simulink model "observer_student"  (R2020b)
settings: Solver=FixedStepAuto  StartTime=0.0  StopTime=Inf  RelTol=1e-3
undefined symbols (not defined in the file): X, Y, Z
libraries: robotlib x12
settings Model: Creator=erlendbasso  LastModifiedBy=erlendbasso
settings OptimizationCC: EnhancedBackFolding=on  PassReuseOutputArgsAs=Individual arguments  ZeroExternalMemoryAtStartup=off  ZeroInternalMemoryAtStartup=off  MaxStackSize=64  OptimizeBlockOrder=speed  DifferentSizesBufferReuse=on  OptimizationCustomize=off  EfficientTunableParamExpr=on
settings DebuggingCC: ParameterTunabilityLossMsg=error
settings HardwareCC: ProdBitPerPointer=32  ProdBitPerSizeT=32  ProdBitPerPtrDiffT=32  ProdLargestAtomicInteger=Long  ProdLargestAtomicFloat=Double  ProdWordSize=32  ProdHWDeviceType=ARM Compatible->ARM Cortex
settings RTWCC: Description=Embedded Coder  SystemTargetFile=ert.tlc  HardwareBoard=Raspberry Pi - Robot Operating System (ROS)  TLCOptions="-aInlineSetEventsForThisBaseRateFcn=TLC_FALSE -aSuppressMultiTaskScheduler=TLC_FALSE  -aRateBasedStepFcn=0"  TemplateMakefile=ert_default_tmf  Toolchain=Catkin  TargetLang=C++
settings CodeAppCC: ForceParamTrailComments=on  IgnoreCustomStorageClasses=off  OperatorAnnotations=on  SimulinkDataObjDesc=on  SFDataObjDesc=on  InsertBlockDesc=on
settings ERTTargetCC: SupportContinuousTime=on  SupportVariableSizeSignals=on

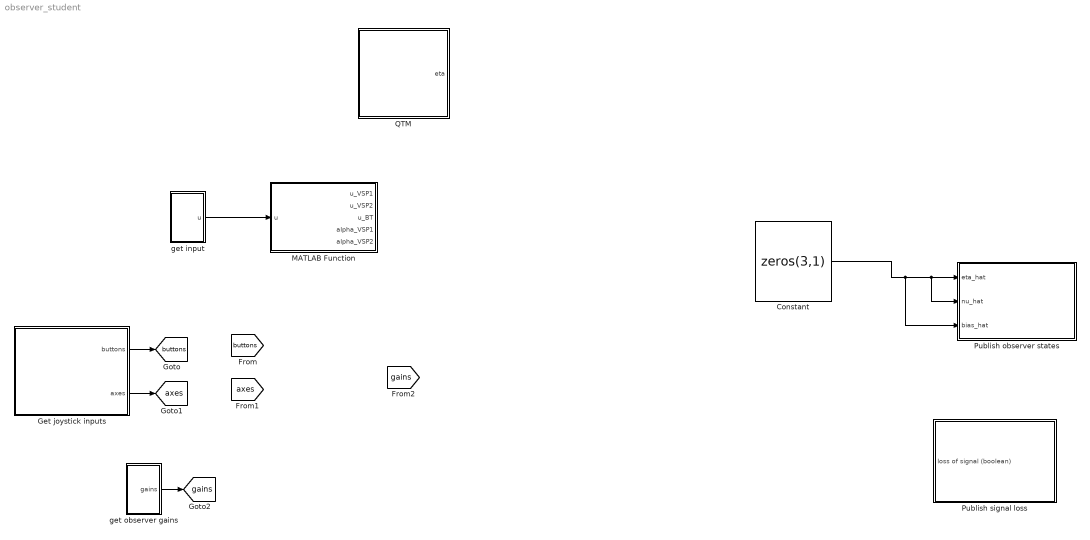
== system observer_student ==
  Constant : Constant  Value=zeros(3,1)
  Get joystick inputs : Subsystem
  MATLAB Function : MATLAB Function  TreatAsAtomicUnit=on
  Publish observer states : Subsystem
  Publish signal loss : Subsystem
  QTM : Subsystem
  get input : Subsystem
  get observer gains : Subsystem
  tag scope: axes=global, buttons=global, gains=global
  wires:
  get input/1(u) -> MATLAB Function/1(u)
  Constant/1 -> Publish observer states/3(bias_hat), Publish observer states/2(nu_hat), Publish observer states/1(eta_hat)
  Get joystick inputs/2(axes) -> [axes]
  Get joystick inputs/1(buttons) -> [buttons]
  get observer gains/1(gains) -> [gains]

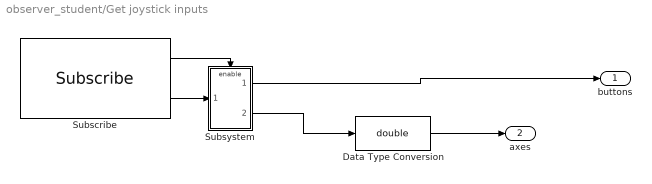
== system observer_student/Get joystick inputs ==
  Data Type Conversion : DataTypeConversion  OutDataTypeStr=double
  Subscribe : robotlib/Subscribe  topicSource=Select from ROS network  topic=/joy  messageType=sensor_msgs/Joy  SampleTime=0.01  legacyBusStruct=off  messageQueueLength=1
  Subsystem : Subsystem
  buttons : Outport
  axes : Outport  Port=2
  wires:
  Subscribe/1 -> Subsystem/Enable
  Subscribe/2 -> Subsystem/1(In1)
  Subsystem/2(<Axes>) -> Data Type Conversion/1
  Subsystem/1(<Buttons>) -> buttons/1
  Data Type Conversion/1 -> axes/1

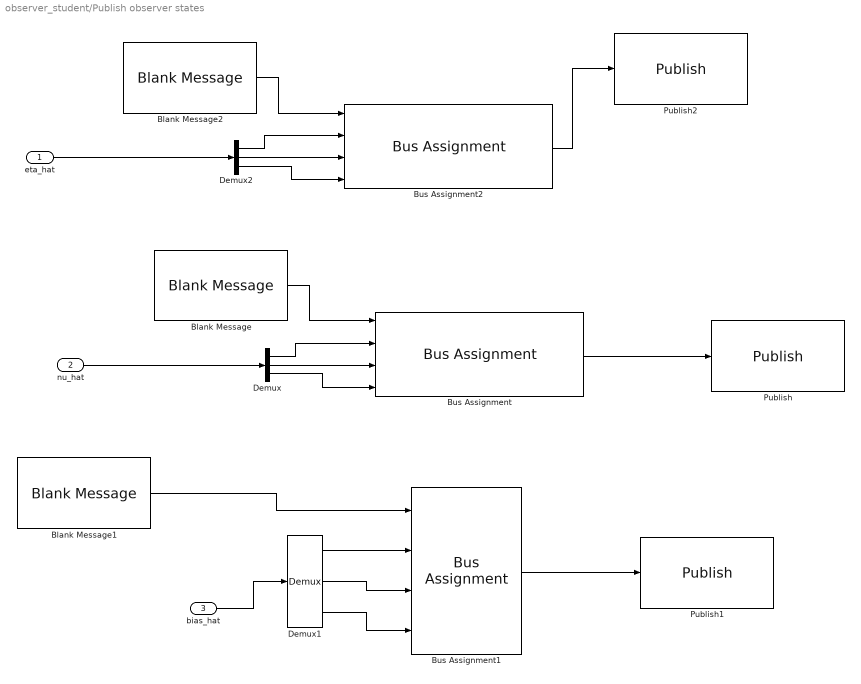
== system observer_student/Publish observer states ==
  eta_hat : Inport
  nu_hat : Inport  Port=2
  bias_hat : Inport  Port=3
  Blank Message : robotlib/Blank Message  messageClass=Message  entityType=geometry_msgs/Vector3  messageType=geometry_msgs/Vector3  SampleTime=0.01  legacyBusStruct=off
  Blank Message1 : robotlib/Blank Message  messageClass=Message  entityType=geometry_msgs/Vector3  messageType=geometry_msgs/Vector3  SampleTime=0.01  legacyBusStruct=off
  Blank Message2 : robotlib/Blank Message  messageClass=Message  entityType=geometry_msgs/Vector3  messageType=geometry_msgs/Vector3  SampleTime=0.01  legacyBusStruct=off
  Bus Assignment : BusAssignment  AssignedSignals=X,Y,Z
  Bus Assignment1 : BusAssignment  AssignedSignals=X,Y,Z
  Bus Assignment2 : BusAssignment  AssignedSignals=X,Y,Z
  Demux : Demux  Outputs=3
  Demux1 : Demux  Outputs=3
  Demux2 : Demux  Outputs=3
  Publish : robotlib/Publish  topicSource=Specify your own  topic=/CSEI/observer/nu  messageType=geometry_msgs/Vector3  legacyBusStruct=off  messageQueueLength=1
  Publish1 : robotlib/Publish  topicSource=Specify your own  topic=/CSEI/observer/bias  messageType=geometry_msgs/Vector3  legacyBusStruct=off  messageQueueLength=1
  Publish2 : robotlib/Publish  topicSource=Specify your own  topic=/CSEI/observer/eta  messageType=geometry_msgs/Vector3  legacyBusStruct=off  messageQueueLength=1
  wires:
  Demux/1 -> Bus Assignment/2
  Bus Assignment/1 -> Publish/1
  nu_hat/1 -> Demux/1
  Demux/2 -> Bus Assignment/3
  Blank Message/1 -> Bus Assignment/1
  Demux/3 -> Bus Assignment/4
  Demux1/2 -> Bus Assignment1/3
  Bus Assignment1/1 -> Publish1/1
  Blank Message1/1 -> Bus Assignment1/1
  Demux1/1 -> Bus Assignment1/2
  Demux1/3 -> Bus Assignment1/4
  bias_hat/1 -> Demux1/1
  eta_hat/1 -> Demux2/1
  Bus Assignment2/1 -> Publish2/1
  Blank Message2/1 -> Bus Assignment2/1
  Demux2/3 -> Bus Assignment2/4
  Demux2/1 -> Bus Assignment2/2
  Demux2/2 -> Bus Assignment2/3

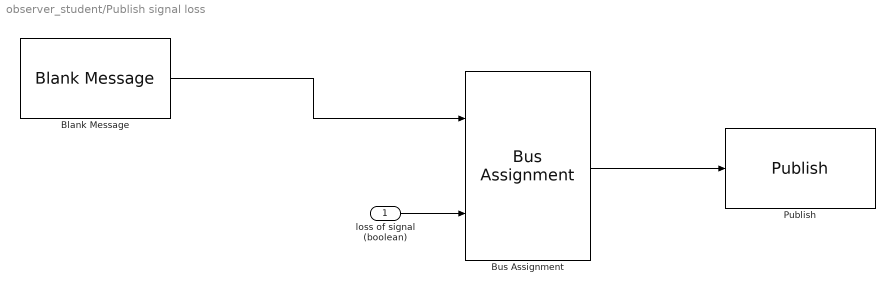
== system observer_student/Publish signal loss ==
  loss of signal (boolean) : Inport  OutDataTypeStr=boolean
  Blank Message : robotlib/Blank Message  messageClass=Message  entityType=std_msgs/Bool  messageType=std_msgs/Bool  SampleTime=0.01  legacyBusStruct=off
  Bus Assignment : BusAssignment  AssignedSignals=Data
  Publish : robotlib/Publish  topicSource=Specify your own  topic=/CSEI/observer/errorsignal  messageType=std_msgs/Bool  legacyBusStruct=off  messageQueueLength=1
  wires:
  Blank Message/1 -> Bus Assignment/1
  Bus Assignment/1 -> Publish/1
  loss of signal (boolean)/1 -> Bus Assignment/2

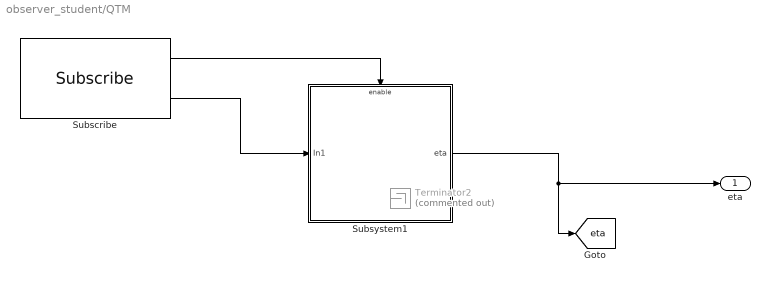
== system observer_student/QTM ==
  Subscribe : robotlib/Subscribe  topicSource=Specify your own  topic=/qualisys/CSEI/odom  messageType=nav_msgs/Odometry  SampleTime=0.01  legacyBusStruct=off  messageQueueLength=1
  Subsystem1 : Subsystem
  Terminator2 : Terminator  Commented=on
  eta : Outport
  tag scope: eta=global
  wires:
  Subscribe/2 -> Subsystem1/1(In1)
  Subscribe/1 -> Subsystem1/Enable
  Subsystem1/1(eta) -> [eta], eta/1

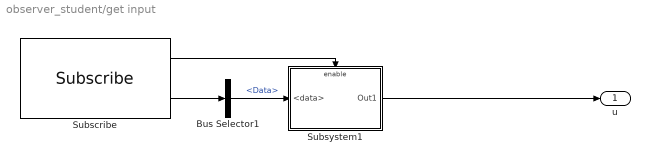
== system observer_student/get input ==
  Bus Selector1 : BusSelector  OutputSignals=Data
  Subscribe : robotlib/Subscribe  topicSource=Specify your own  topic=/CSEI/u  messageType=std_msgs/Float64MultiArray  SampleTime=0.01  legacyBusStruct=off  messageQueueLength=1
  Subsystem1 : Subsystem
  u : Outport
  wires:
  Subscribe/1 -> Subsystem1/Enable
  Subscribe/2 -> Bus Selector1/1
  Subsystem1/1(Out1) -> u/1
  Bus Selector1/1 -> Subsystem1/1(<data>)  "<Data>"

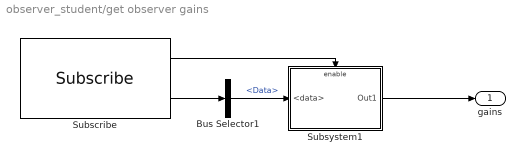
== system observer_student/get observer gains ==
  Bus Selector1 : BusSelector  OutputSignals=Data
  Subscribe : robotlib/Subscribe  topicSource=Specify your own  topic=/CSEI/observer/gains  messageType=std_msgs/Float64MultiArray  SampleTime=0.01  legacyBusStruct=off  messageQueueLength=1
  Subsystem1 : Subsystem
  gains : Outport
  wires:
  Subsystem1/1(Out1) -> gains/1
  Subscribe/1 -> Subsystem1/Enable
  Subscribe/2 -> Bus Selector1/1
  Bus Selector1/1 -> Subsystem1/1(<data>)  "<Data>"

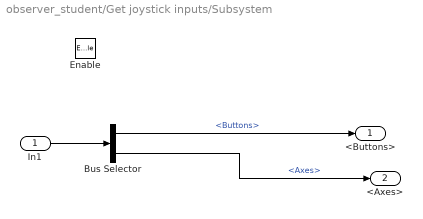
== system observer_student/Get joystick inputs/Subsystem ==
  In1 : Inport
  Enable : EnablePort
  Bus Selector : BusSelector  OutputSignals=Buttons,Axes
  <Buttons> : Outport
  <Axes> : Outport  Port=2
  wires:
  In1/1 -> Bus Selector/1
  Bus Selector/1 -> <Buttons>/1  "<Buttons>"
  Bus Selector/2 -> <Axes>/1  "<Axes>"

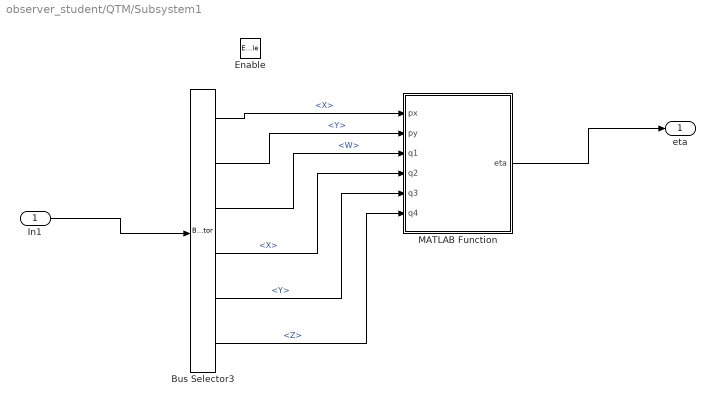
== system observer_student/QTM/Subsystem1 ==
  In1 : Inport
  Enable : EnablePort
  Bus Selector3 : BusSelector  OutputSignals=Pose.Pose.Position.X,Pose.Pose.Position.Y,Pose.Pose.Orientation.W,Pose.Pose.Orientation.X,Pose.Pose.Orientation.Y,Pose.Pose.Orientation.Z
  MATLAB Function : MATLAB Function  TreatAsAtomicUnit=on
  eta : Outport
  wires:
  In1/1 -> Bus Selector3/1
  MATLAB Function/1(eta) -> eta/1
  Bus Selector3/1 -> MATLAB Function/1(px)  "<X>"
  Bus Selector3/2 -> MATLAB Function/2(py)  "<Y>"
  Bus Selector3/3 -> MATLAB Function/3(q1)  "<W>"
  Bus Selector3/4 -> MATLAB Function/4(q2)  "<X>"
  Bus Selector3/5 -> MATLAB Function/5(q3)  "<Y>"
  Bus Selector3/6 -> MATLAB Function/6(q4)  "<Z>"

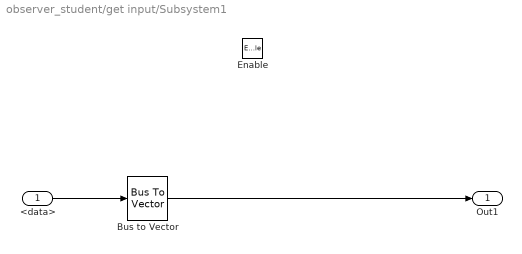
== system observer_student/get input/Subsystem1 ==
  <data> : Inport
  Enable : EnablePort
  Bus to Vector : BusToVector
  Out1 : Outport
  wires:
  Bus to Vector/1 -> Out1/1
  <data>/1 -> Bus to Vector/1

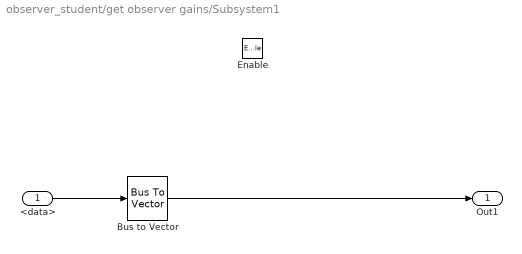
== system observer_student/get observer gains/Subsystem1 ==
  <data> : Inport
  Enable : EnablePort
  Bus to Vector : BusToVector
  Out1 : Outport
  wires:
  Bus to Vector/1 -> Out1/1
  <data>/1 -> Bus to Vector/1

== matlab function observer_student/MATLAB Function ==
  data: u_VSP1 output; u_VSP2 output; u input; u_BT output; alpha_VSP1 output; alpha_VSP2 output
function [u_VSP1,u_VSP2,u_BT,alpha_VSP1,alpha_VSP2] = fcn(u)
u_VSP1 = u(1);
u_VSP2 = u(2);
u_BT = u(3);
alpha_VSP1 = u(4);
alpha_VSP2 = u(5);

== matlab function observer_student/QTM/Subsystem1/MATLAB Function ==
  data: px input; eta output; py input; q1 input; q2 input; q3 input; q4 input
function eta = fcn(px,py,q1,q2,q3,q4)

quat = [q1;q2;q3;q4];
eul = quat2eul(quat','XYZ');

eta = [px;py;eul(3)];
